simulink model "simulink5ms_plotAndGains"  (R2018a)
settings: Solver=ode3  StartTime=0.0  StopTime=35  FixedStep=.005  RelTol=1e-3  EnableMultiTasking=on
StartFcn:
  | set_toolbars_for_model(gcs,'off');
StopFcn:
  | set_toolbars_for_model(gcs,'on');
undefined symbols (not defined in the file or in its folder): Serial_Port, Standard_Devices
libraries: sldrtlib x2
settings Model: SimulationMode=external  ExtModeTrigDuration=10000  Creator=d-block  LastModifiedBy=ayush2
settings DataIOCC: LimitDataPoints=on  SaveFormat=Array
settings OptimizationCC: LifeSpan=inf
settings DebuggingCC: SFUnexpectedBacktrackingDiag=warning  SFNoUnconditionalDefaultTransitionDiag=warning  SFExecutionAtInitializationDiag=none
settings HardwareCC: TargetBitPerLong=64  TargetBitPerPointer=64  TargetIntDivRoundTo=Zero  TargetEndianess=LittleEndian  TargetWordSize=64  TargetHWDeviceType=Intel->x86-64
settings ModelReferenceCC: PropagateSignalLabelsOutOfModel=off
settings RTWCC: SystemTargetFile=sldrt.tlc  TemplateMakefile=sldrt.tmf  Description=Simulink Desktop Real-Time  RTWCompilerOptimization=on
settings CodeAppCC: MaxIdLength=95  StateflowObjectComments=on
settings SimulinkDesktopRealTimeCC: TargetPreCompLibLocation=C:\MATLABR2018a\toolbox\sldrt\lib\win64  TargetLangStandard=C89/C90 (ANSI)  SupportVariableSizeSignals=off
settings ConfigComp: CovMetricSettings=dw  CovHtmlReporting=on  CovSaveCumulativeToWorkspaceVar=on  CovSaveSingleToWorkspaceVar=on  CovExternalEMLEnable=off

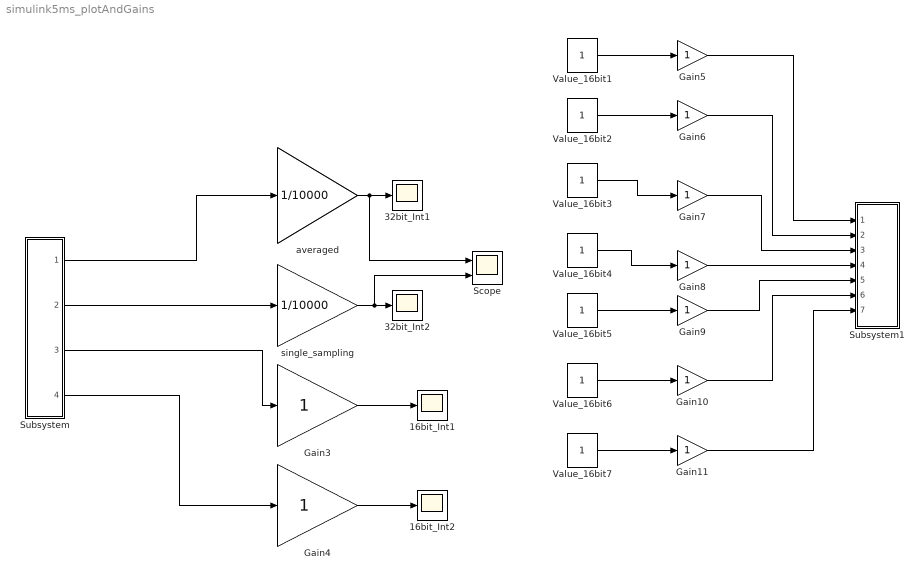
== system simulink5ms_plotAndGains ==
  16bit_Int1 : Scope
  16bit_Int2 : Scope
  32bit_Int1 : Scope
  32bit_Int2 : Scope
  Gain{5..11} (7 alike) : Gain
  Gain3 : Gain  OutDataTypeStr=double  SaturateOnIntegerOverflow=on  ParamDataTypeStr=Inherit: Same as input
  Gain4 : Gain  OutDataTypeStr=double  SaturateOnIntegerOverflow=on  ParamDataTypeStr=Inherit: Same as input
  Scope : Scope  NumInputPorts=2
  Subsystem : Subsystem
  Subsystem1 : Subsystem
  Value_16bit{1..4,6..7} (6 alike) : Constant
  "Value_16bit5 " : Constant
  averaged : Gain  Gain=1/10000  OutDataTypeStr=double  SaturateOnIntegerOverflow=on  ParamDataTypeStr=Inherit: Same as input
  single_sampling : Gain  Gain=1/10000  OutDataTypeStr=double  SaturateOnIntegerOverflow=on  ParamDataTypeStr=Inherit: Same as input
  wires:
  Subsystem/1(32bit_Int1) -> averaged/1
  single_sampling/1 -> Scope/2, 32bit_Int2/1
  Value_16bit2/1 -> Gain6/1
  Value_16bit3/1 -> Gain7/1
  Value_16bit4/1 -> Gain8/1
  "Value_16bit5 "/1 -> Gain9/1
  Subsystem/3(16bit_Int1) -> Gain3/1
  Subsystem/4(16bit_Int2) -> Gain4/1
  Subsystem/2(32bit_Int2) -> single_sampling/1
  Gain3/1 -> 16bit_Int1/1
  Gain4/1 -> 16bit_Int2/1
  Value_16bit1/1 -> Gain5/1
  Value_16bit6/1 -> Gain10/1
  Value_16bit7/1 -> Gain11/1
  averaged/1 -> Scope/1, 32bit_Int1/1
  Gain5/1 -> Subsystem1/1(Data1)
  Gain6/1 -> Subsystem1/2(Data2)
  Gain7/1 -> Subsystem1/3(Data3)
  Gain8/1 -> Subsystem1/4(Data4)
  Gain9/1 -> Subsystem1/5(Data5)
  Gain10/1 -> Subsystem1/6("Data6 ")
  Gain11/1 -> Subsystem1/7("Data7 ")

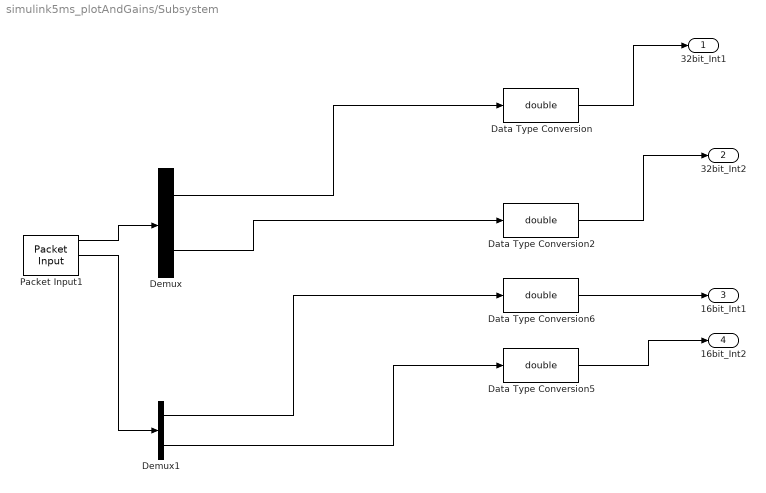
== system simulink5ms_plotAndGains/Subsystem ==
  Data Type Conversion{,2,5..6} (4 alike) : DataTypeConversion  OutDataTypeStr=double
  Demux : Demux  Outputs=2
  Demux1 : Demux  Outputs=2
  Packet Input1 : sldrtlib/Packet Input  SampleTime=.005  MaxMissedTicks=50  ShowMissedTicks=on  YieldWhenWaiting=off  DrvName=Standard_Devices/Serial_Port  DrvAddress=1  DrvOptions=[115200 8 0 0 0 0 0 1]  PacketSize=12  DataTypes={'2*int32','2*int16'}  ShowReady=off  ShowError=off  PacketID=1  ByteOrder=1  ShowTimestamp=off
      settings: AttributesFormatString=Standard Devices\nSerial Port [1h]  SourceProductName=Simulink Desktop Real-Time
  32bit_Int1 : Outport
  32bit_Int2 : Outport  Port=2
  16bit_Int1 : Outport  Port=3
  16bit_Int2 : Outport  Port=4
  wires:
  Data Type Conversion/1 -> 32bit_Int1/1
  Data Type Conversion2/1 -> 32bit_Int2/1
  Data Type Conversion6/1 -> 16bit_Int1/1
  Data Type Conversion5/1 -> 16bit_Int2/1
  Demux1/2 -> Data Type Conversion5/1
  Demux1/1 -> Data Type Conversion6/1
  Packet Input1/1 -> Demux/1
  Packet Input1/2 -> Demux1/1
  Demux/1 -> Data Type Conversion/1
  Demux/2 -> Data Type Conversion2/1

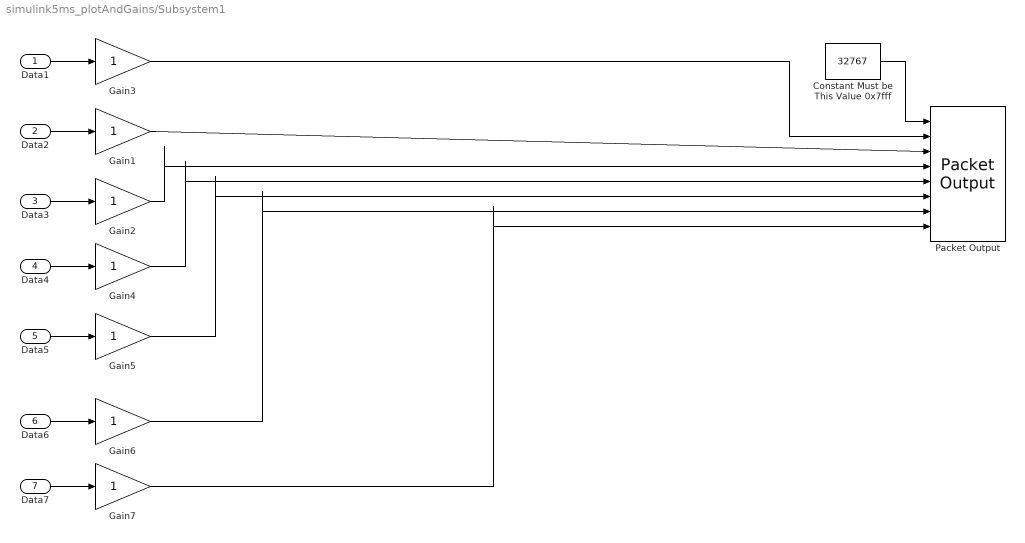
== system simulink5ms_plotAndGains/Subsystem1 ==
  Data1 : Inport
  Data2 : Inport  Port=2
  Data3 : Inport  Port=3
  Data4 : Inport  Port=4
  Data5 : Inport  Port=5
  "Data6 " : Inport  Port=6
  "Data7 " : Inport  Port=7
  Constant Must be This Value 0x7fff : Constant  Value=32767  OutDataTypeStr=int16
  Gain{1..7} (7 alike) : Gain  OutDataTypeStr=int16
  Packet Output : sldrtlib/Packet Output  SampleTime=.005  MaxMissedTicks=10  ShowMissedTicks=off  YieldWhenWaiting=off  DrvName=Standard_Devices/Serial_Port  DrvAddress=1  DrvOptions=[115200 8 0 0 0 0 0 1]  PacketSize=16  DataTypes={'int16','int16','int16','int16','int16','int16','int16','int16'}  ShowReady=off  ShowError=off  PacketID=1  ByteOrder=1  InitialValue=[]  FinalValue=[]
      settings: AttributesFormatString=Standard Devices\nSerial Port [1h]  SourceProductName=Simulink Desktop Real-Time
  wires:
  Data1/1 -> Gain3/1
  Data2/1 -> Gain1/1
  Data3/1 -> Gain2/1
  Data5/1 -> Gain5/1
  Gain3/1 -> Packet Output/2
  Data4/1 -> Gain4/1
  "Data6 "/1 -> Gain6/1
  "Data7 "/1 -> Gain7/1
  Constant Must be This Value 0x7fff/1 -> Packet Output/1
  Gain1/1 -> Packet Output/3
  Gain2/1 -> Packet Output/4
  Gain4/1 -> Packet Output/5
  Gain5/1 -> Packet Output/6
  Gain6/1 -> Packet Output/7
  Gain7/1 -> Packet Output/8
